simulink model "Quiz2_A"  (R2023a)
settings: Solver=VariableStepAuto  StartTime=0.0  StopTime=40  RelTol=1e-3
settings Model: Creator=massey_andrew  LastModifiedBy=massey_andrew

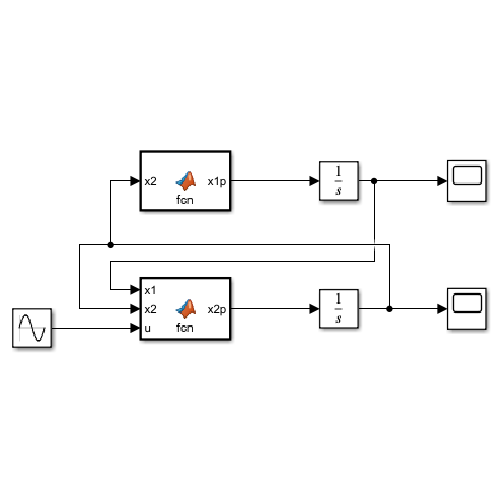
[thumbnail: Simulink's stored preview of the top-level diagram]
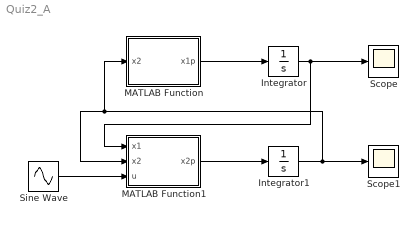
== system Quiz2_A ==
  Integrator : Integrator
  Integrator1 : Integrator
  MATLAB Function : MATLAB Function  TreatAsAtomicUnit=on
  MATLAB Function1 : MATLAB Function  TreatAsAtomicUnit=on
  Scope : Scope
  Scope1 : Scope
  Sine Wave : Sin  Amplitude=1.2  Frequency=(2*pi)/10  SampleTime=0
  wires:
  MATLAB Function/1(x1p) -> Integrator/1
  Sine Wave/1 -> MATLAB Function1/3(u)
  MATLAB Function1/1(x2p) -> Integrator1/1
  Integrator/1 -> Scope/1, MATLAB Function1/1(x1)
  Integrator1/1 -> Scope1/1, MATLAB Function1/2(x2), MATLAB Function/1(x2)

== matlab function Quiz2_A/MATLAB Function ==
  data: x2 input; x1p output
function x1p = fcn(x2)

x1p = x2;

== matlab function Quiz2_A/MATLAB Function1 ==
  data: x1 input; x2 input; x2p output; u input
function x2p = fcn(x1,x2,u)

mu = 8.53;

x2p = mu*(1-x1^2)*x2-x1+u;
